simulink model "MEMS_Gyro_Structure_Model"  (R2019b)
settings: Solver=VariableStepAuto  StartTime=0.0  StopTime=10.0  RelTol=1e-3
settings Model: Creator=Rio  LastModifiedBy=Rio

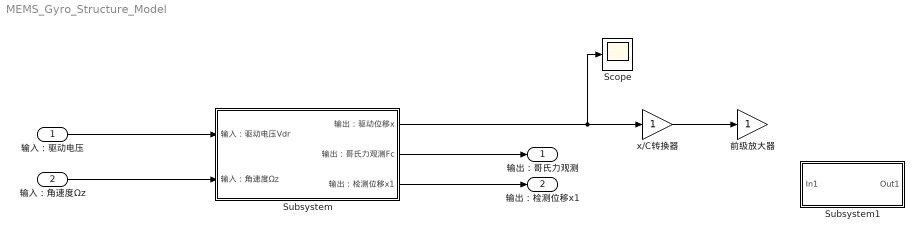
== system MEMS_Gyro_Structure_Model ==
  输入：驱动电压 : Inport
  输入：角速度Ωz : Inport  Port=2
  Scope : Scope
  Subsystem : Subsystem
  Subsystem1 : Subsystem
  x/C转换器 : Gain
  前级放大器 : Gain
  输出：哥氏力观测 : Outport
  输出：检测位移x1 : Outport  Port=2
  wires:
  输入：驱动电压/1 -> Subsystem/1(输入：驱动电压Vdr)
  输入：角速度Ωz/1 -> Subsystem/2(输入：角速度Ωz)
  Subsystem/1(输出：驱动位移x) -> Scope/1, x/C转换器/1
  Subsystem/2(输出：哥氏力观测Fc) -> 输出：哥氏力观测/1
  Subsystem/3(输出：检测位移x1) -> 输出：检测位移x1/1
  x/C转换器/1 -> 前级放大器/1

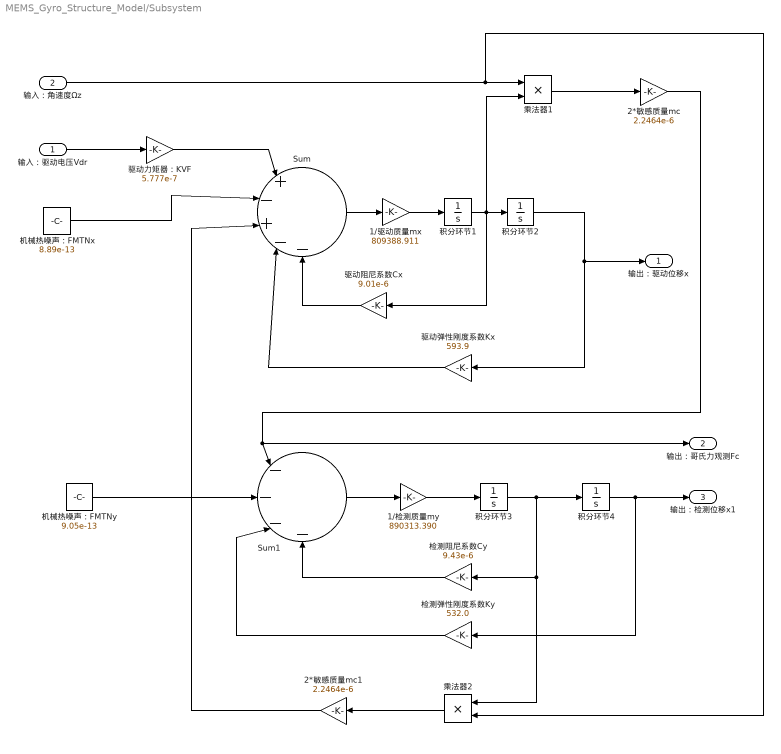
== system MEMS_Gyro_Structure_Model/Subsystem ==
  输入：驱动电压Vdr : Inport
  输入：角速度Ωz : Inport  Port=2
  1/检测质量my : Gain  Gain=890313.390
  1/驱动质量mx : Gain  Gain=809388.911
  2*敏感质量mc : Gain  Gain=2.2464e-6
  2*敏感质量mc1 : Gain  Gain=2.2464e-6
  Sum : Sum  Inputs=|+-+--
  Sum1 : Sum  Inputs=|----
  乘法器1 : Product
  乘法器2 : Product
  机械热噪声：FMTNx : Constant  Value=8.89e-13
  机械热噪声：FMTNy : Constant  Value=9.05e-13
  检测弹性刚度系数Ky : Gain  Gain=532.0
  检测阻尼系数Cy : Gain  Gain=9.43e-6
  积分环节{1..4} (4 alike) : Integrator
  驱动力矩器：KVF : Gain  Gain=5.777e-7
  驱动弹性刚度系数Kx : Gain  Gain=593.9
  驱动阻尼系数Cx : Gain  Gain=9.01e-6
  输出：驱动位移x : Outport
  输出：哥氏力观测Fc : Outport  Port=2
  输出：检测位移x1 : Outport  Port=3
  wires:
  1/检测质量my/1 -> 积分环节3/1
  积分环节1/1 -> 驱动阻尼系数Cx/1, 乘法器1/2, 积分环节2/1
  积分环节4/1 -> 输出：检测位移x1/1, 检测弹性刚度系数Ky/1
  机械热噪声：FMTNx/1 -> Sum/2
  2*敏感质量mc/1 -> 输出：哥氏力观测Fc/1, Sum1/1
  积分环节3/1 -> 乘法器2/1, 检测阻尼系数Cy/1, 积分环节4/1
  检测弹性刚度系数Ky/1 -> Sum1/3
  Sum1/1 -> 1/检测质量my/1
  输入：驱动电压Vdr/1 -> 驱动力矩器：KVF/1
  机械热噪声：FMTNy/1 -> Sum1/2
  积分环节2/1 -> 输出：驱动位移x/1, 驱动弹性刚度系数Kx/1
  输入：角速度Ωz/1 -> 乘法器2/2, 乘法器1/1
  Sum/1 -> 1/驱动质量mx/1
  驱动阻尼系数Cx/1 -> Sum/5
  2*敏感质量mc1/1 -> Sum/3
  驱动弹性刚度系数Kx/1 -> Sum/4
  乘法器1/1 -> 2*敏感质量mc/1
  驱动力矩器：KVF/1 -> Sum/1
  1/驱动质量mx/1 -> 积分环节1/1
  乘法器2/1 -> 2*敏感质量mc1/1
  检测阻尼系数Cy/1 -> Sum1/4

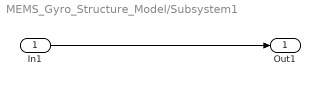
== system MEMS_Gyro_Structure_Model/Subsystem1 ==
  In1 : Inport
  Out1 : Outport
  wires:
  In1/1 -> Out1/1
